simulink model "Quadcopter"  (R2022b)
settings: Solver=FixedStepAuto  StartTime=0.0  StopTime=sim_time  FixedStep=step_size  RelTol=1e-3
undefined symbols (not defined in the file or in its folder): gain, init
settings Model: Creator=Sebastian  LastModifiedBy=Sebastian

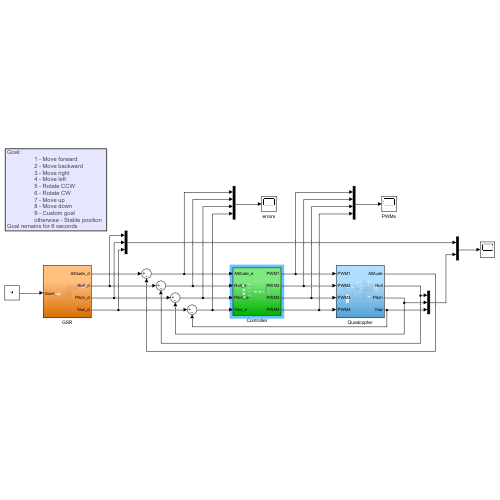
[thumbnail: Simulink's stored preview of the top-level diagram]
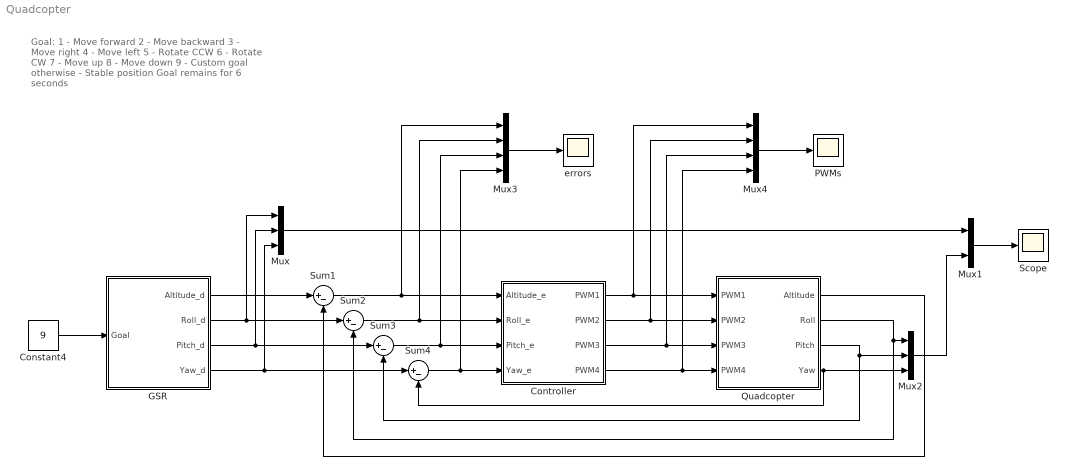
== system Quadcopter ==
  note: Goal:
      |                  1 - Move forward
      |                  2 - Move backward
      |                  3 - Move right
      |                  4 - Move left
      |                  5 - Rotate CCW
      |                  6 - Rotate CW
      |                  7 - Move up
      |                  8 - Move down
      |                  9 - Custom goal
      |                  otherwise - Stable position
      | Goal remains for 6 seconds
  Constant4 : Constant  Value=9
  Controller : Subsystem
  GSR : Subsystem
  Mux : Mux  Inputs=3
  Mux1 : Mux  Inputs=2
  Mux2 : Mux  Inputs=3
  Mux3 : Mux
  Mux4 : Mux
  PWMs : Scope
  Quadcopter : Subsystem
  Scope : Scope
  Sum{1..4} (4 alike) : Sum  Inputs=|+-
  errors : Scope
  wires:
  Constant4/1 -> GSR/1(Goal)
  GSR/2(Roll_d) -> Mux/1, Sum2/1
  Quadcopter/2(Roll) -> Sum2/2, Mux2/1
  GSR/3(Pitch_d) -> Mux/2, Sum3/1
  GSR/4(Yaw_d) -> Mux/3, Sum4/1
  Quadcopter/3(Pitch) -> Sum3/2, Mux2/2
  Quadcopter/4(Yaw) -> Mux2/3, Sum4/2
  Sum2/1 -> Mux3/2, Controller/2(Roll_e)
  Sum3/1 -> Mux3/3, Controller/3(Pitch_e)
  Sum4/1 -> Controller/4(Yaw_e), Mux3/4
  Mux/1 -> Mux1/1
  Mux2/1 -> Mux1/2
  Mux1/1 -> Scope/1
  Quadcopter/1(Altitude) -> Sum1/2
  GSR/1(Altitude_d) -> Sum1/1
  Sum1/1 -> Mux3/1, Controller/1(Altitude_e)
  Controller/1(PWM1) -> Mux4/1, Quadcopter/1(PWM1)
  Controller/2(PWM2) -> Mux4/2, Quadcopter/2(PWM2)
  Controller/3(PWM3) -> Mux4/3, Quadcopter/3(PWM3)
  Controller/4(PWM4) -> Mux4/4, Quadcopter/4(PWM4)
  Mux3/1 -> errors/1
  Mux4/1 -> PWMs/1

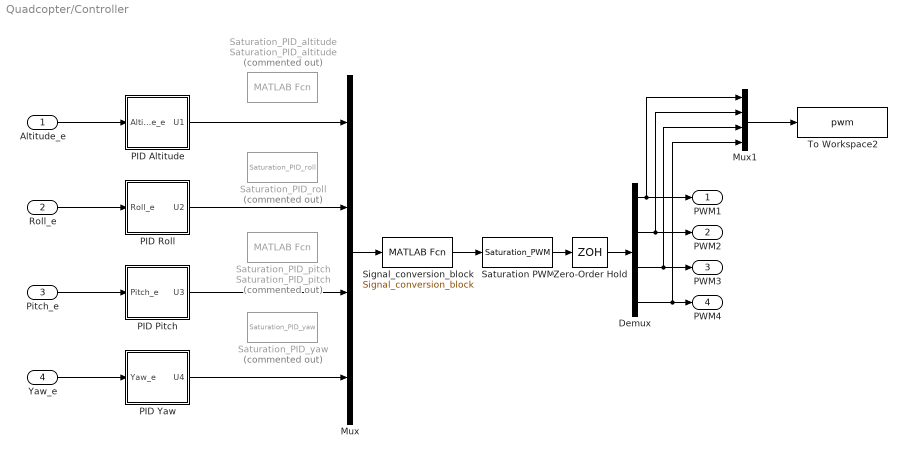
== system Quadcopter/Controller ==
  Altitude_e : Inport
  Roll_e : Inport  Port=2
  Pitch_e : Inport  Port=3
  Yaw_e : Inport  Port=4
  Demux : Demux
  Mux : Mux
  Mux1 : Mux
  PID Altitude : Subsystem
  PID Pitch : Subsystem
  PID Roll : Subsystem
  PID Yaw : Subsystem
  Saturation PWM : MATLABFcn  MATLABFcn=Saturation_PWM  OutputDimensions=4
  Saturation_PID_altitude : MATLABFcn  Commented=on  MATLABFcn=Saturation_PID_altitude  OutputDimensions=1
  Saturation_PID_pitch : MATLABFcn  Commented=on  MATLABFcn=Saturation_PID_pitch  OutputDimensions=1
  Saturation_PID_roll : MATLABFcn  Commented=on  MATLABFcn=Saturation_PID_roll  OutputDimensions=1
  Saturation_PID_yaw : MATLABFcn  Commented=on  MATLABFcn=Saturation_PID_yaw  OutputDimensions=1
  Signal_conversion_block : MATLABFcn  MATLABFcn=Signal_conversion_block  OutputDimensions=4
  To Workspace2 : ToWorkspace  VariableName=pwm  SampleTime=-1
  Zero-Order Hold : ZeroOrderHold  SampleTime=-1
  PWM1 : Outport
  PWM2 : Outport  Port=2
  PWM3 : Outport  Port=3
  PWM4 : Outport  Port=4
  wires:
  Mux/1 -> Signal_conversion_block/1
  Signal_conversion_block/1 -> Saturation PWM/1
  Demux/1 -> Mux1/1, PWM1/1
  Demux/3 -> Mux1/3, PWM3/1
  Roll_e/1 -> PID Roll/1(Roll_e)
  Demux/2 -> Mux1/2, PWM2/1
  Demux/4 -> Mux1/4, PWM4/1
  Yaw_e/1 -> PID Yaw/1(Yaw_e)
  PID Yaw/1(U4) -> Mux/4
  Pitch_e/1 -> PID Pitch/1(Pitch_e)
  PID Pitch/1(U3) -> Mux/3
  PID Roll/1(U2) -> Mux/2
  Altitude_e/1 -> PID Altitude/1(Altitude_e)
  PID Altitude/1(U1) -> Mux/1
  Mux1/1 -> To Workspace2/1
  Saturation PWM/1 -> Zero-Order Hold/1
  Zero-Order Hold/1 -> Demux/1

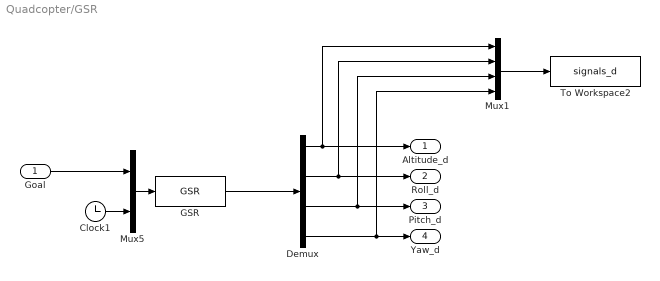
== system Quadcopter/GSR ==
  Goal : Inport
  Clock1 : Clock
  Demux : Demux
  GSR : MATLABFcn  MATLABFcn=GSR  OutputDimensions=4
  Mux1 : Mux
  Mux5 : Mux  Inputs=2
  To Workspace2 : ToWorkspace  VariableName=signals_d  SampleTime=-1
  Altitude_d : Outport
  Roll_d : Outport  Port=2
  Pitch_d : Outport  Port=3
  Yaw_d : Outport  Port=4
  wires:
  Demux/1 -> Mux1/1, Altitude_d/1
  Demux/4 -> Mux1/4, Yaw_d/1
  Mux5/1 -> GSR/1
  Goal/1 -> Mux5/1
  Demux/2 -> Mux1/2, Roll_d/1
  Clock1/1 -> Mux5/2
  Demux/3 -> Mux1/3, Pitch_d/1
  Mux1/1 -> To Workspace2/1
  GSR/1 -> Demux/1

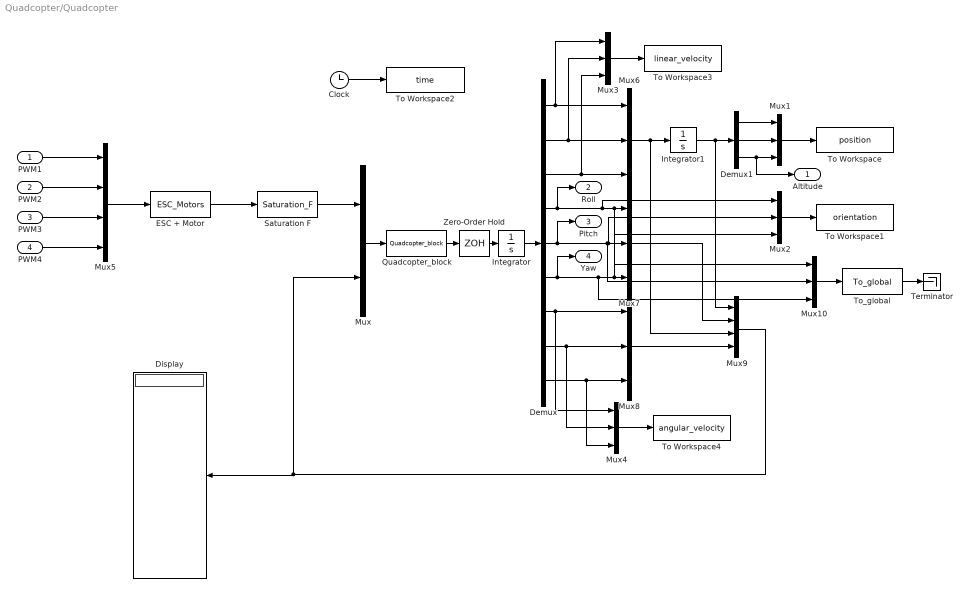
== system Quadcopter/Quadcopter ==
  PWM1 : Inport
  PWM2 : Inport  Port=2
  PWM3 : Inport  Port=3
  PWM4 : Inport  Port=4
  Clock : Clock
  Demux : Demux  Outputs=9
  Demux1 : Demux  Outputs=3
  Display : Display
  ESC + Motor : MATLABFcn  MATLABFcn=ESC_Motors  OutputDimensions=4
  Integrator : Integrator  InitialCondition=[init.dx init.dy init.dz init.phi init.theta init.psi init.p init.q init.r]
  Integrator1 : Integrator  InitialCondition=[init.x init.y init.z]
  Mux : Mux  Inputs=2
  Mux{1..4,6..8,10} (8 alike) : Mux  Inputs=3
  Mux5 : Mux
  Mux9 : Mux
  Quadcopter_block : MATLABFcn  MATLABFcn=Quadcopter_block  OutputDimensions=9
  Saturation F : MATLABFcn  MATLABFcn=Saturation_F  OutputDimensions=4
  Terminator : Terminator
  To Workspace : ToWorkspace  VariableName=position  SampleTime=-1
  To Workspace1 : ToWorkspace  VariableName=orientation  SampleTime=-1
  To Workspace2 : ToWorkspace  VariableName=time  SampleTime=-1
  To Workspace3 : ToWorkspace  VariableName=linear_velocity  SampleTime=-1
  To Workspace4 : ToWorkspace  VariableName=angular_velocity  SampleTime=-1
  To_global : MATLABFcn  MATLABFcn=To_global  OutputDimensions=1
  Zero-Order Hold : ZeroOrderHold  SampleTime=-1
  Altitude : Outport
  Roll : Outport  Port=2
  Pitch : Outport  Port=3
  Yaw : Outport  Port=4
  wires:
  Demux1/2 -> Mux1/2
  Integrator1/1 -> Mux9/1, Demux1/1
  Demux/2 -> Mux3/2, Mux6/2
  Demux/8 -> Mux4/2, Mux8/2
  Demux/3 -> Mux6/3, Mux3/3
  Demux/4 -> Roll/1, Mux10/1, Mux7/1, Mux2/1
  Mux/1 -> Quadcopter_block/1
  Demux/5 -> Pitch/1, Mux10/2, Mux7/2, Mux2/2
  Demux/1 -> Mux6/1, Mux3/1
  Demux1/3 -> Altitude/1, Mux1/3
  Demux1/1 -> Mux1/1
  Mux4/1 -> To Workspace4/1
  Mux1/1 -> To Workspace/1
  Demux/6 -> Yaw/1, Mux10/3, Mux7/3, Mux2/3
  Mux2/1 -> To Workspace1/1
  Mux3/1 -> To Workspace3/1
  Clock/1 -> To Workspace2/1
  PWM1/1 -> Mux5/1
  Demux/7 -> Mux4/1, Mux8/1
  Mux8/1 -> Mux9/4
  Mux7/1 -> Mux9/2
  Mux9/1 -> Mux/2, Display/1
  Mux6/1 -> Mux9/3, Integrator1/1
  Demux/9 -> Mux4/3, Mux8/3
  PWM4/1 -> Mux5/4
  Saturation F/1 -> Mux/1
  Integrator/1 -> Demux/1
  PWM2/1 -> Mux5/2
  PWM3/1 -> Mux5/3
  To_global/1 -> Terminator/1
  Mux10/1 -> To_global/1
  ESC + Motor/1 -> Saturation F/1
  Mux5/1 -> ESC + Motor/1
  Quadcopter_block/1 -> Zero-Order Hold/1
  Zero-Order Hold/1 -> Integrator/1

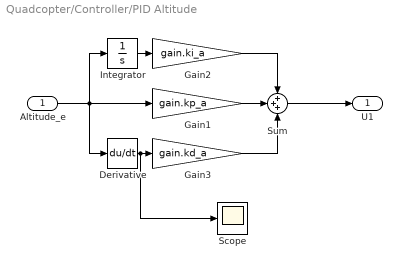
== system Quadcopter/Controller/PID Altitude ==
  Altitude_e : Inport
  Derivative : Derivative
  Gain1 : Gain  Gain=gain.kp_a
  Gain2 : Gain  Gain=gain.ki_a
  Gain3 : Gain  Gain=gain.kd_a
  Integrator : Integrator
  Scope : Scope
  Sum : Sum  Inputs=+++
  U1 : Outport
  wires:
  Gain1/1 -> Sum/2
  Sum/1 -> U1/1
  Derivative/1 -> Scope/1, Gain3/1
  Integrator/1 -> Gain2/1
  Gain3/1 -> Sum/3
  Gain2/1 -> Sum/1
  Altitude_e/1 -> Gain1/1, Integrator/1, Derivative/1

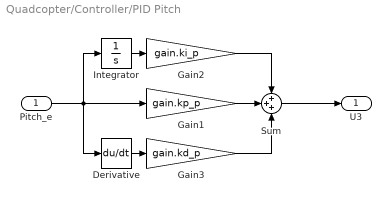
== system Quadcopter/Controller/PID Pitch ==
  Pitch_e : Inport
  Derivative : Derivative
  Gain1 : Gain  Gain=gain.kp_p
  Gain2 : Gain  Gain=gain.ki_p
  Gain3 : Gain  Gain=gain.kd_p
  Integrator : Integrator
  Sum : Sum  Inputs=+++
  U3 : Outport
  wires:
  Pitch_e/1 -> Derivative/1, Integrator/1, Gain1/1
  Gain1/1 -> Sum/2
  Derivative/1 -> Gain3/1
  Sum/1 -> U3/1
  Integrator/1 -> Gain2/1
  Gain3/1 -> Sum/3
  Gain2/1 -> Sum/1

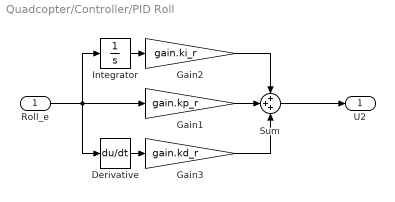
== system Quadcopter/Controller/PID Roll ==
  Roll_e : Inport
  Derivative : Derivative
  Gain1 : Gain  Gain=gain.kp_r
  Gain2 : Gain  Gain=gain.ki_r
  Gain3 : Gain  Gain=gain.kd_r
  Integrator : Integrator
  Sum : Sum  Inputs=+++
  U2 : Outport
  wires:
  Roll_e/1 -> Derivative/1, Integrator/1, Gain1/1
  Gain2/1 -> Sum/1
  Gain3/1 -> Sum/3
  Integrator/1 -> Gain2/1
  Derivative/1 -> Gain3/1
  Sum/1 -> U2/1
  Gain1/1 -> Sum/2

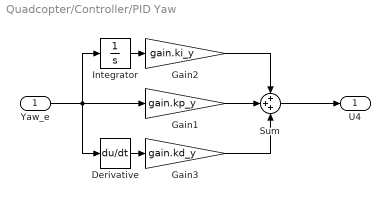
== system Quadcopter/Controller/PID Yaw ==
  Yaw_e : Inport
  Derivative : Derivative
  Gain1 : Gain  Gain=gain.kp_y
  Gain2 : Gain  Gain=gain.ki_y
  Gain3 : Gain  Gain=gain.kd_y
  Integrator : Integrator
  Sum : Sum  Inputs=+++
  U4 : Outport
  wires:
  Yaw_e/1 -> Derivative/1, Integrator/1, Gain1/1
  Gain1/1 -> Sum/2
  Derivative/1 -> Gain3/1
  Sum/1 -> U4/1
  Integrator/1 -> Gain2/1
  Gain3/1 -> Sum/3
  Gain2/1 -> Sum/1
